simulink model "temperature_controller"  (R2026a)
settings: Solver=FixedStepDiscrete  StopTime=0  FixedStep=1
libraries: simulink x2
settings Model: Creator=Nouran Ismail  LastModifiedBy=Nouran Ismail

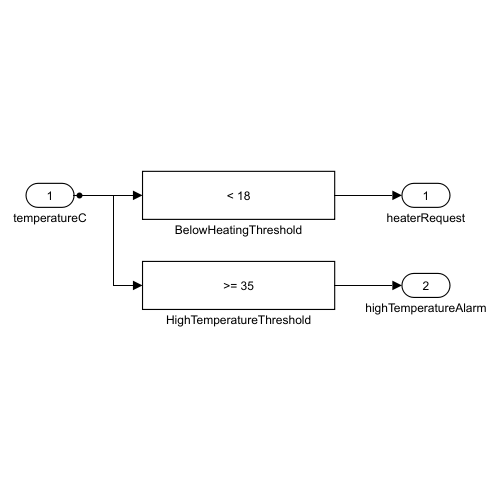
[thumbnail: Simulink's stored preview of the top-level diagram]
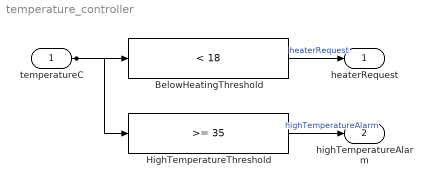
== system temperature_controller ==
  temperatureC : Inport  OutDataTypeStr=double
  BelowHeatingThreshold : simulink/Logic and Bit Operations/Compare To Constant  relop=<  const=18  OutDataTypeStr=boolean
  HighTemperatureThreshold : simulink/Logic and Bit Operations/Compare To Constant  relop=>=  const=35  OutDataTypeStr=boolean
  heaterRequest : Outport
  highTemperatureAlarm : Outport  Port=2
  wires:
  temperatureC/1 -> BelowHeatingThreshold/1, HighTemperatureThreshold/1
  BelowHeatingThreshold/1 -> heaterRequest/1  "heaterRequest"
  HighTemperatureThreshold/1 -> highTemperatureAlarm/1  "highTemperatureAlarm"
